simulink model "Test_N4"  (R2020b)
settings: Solver=ode3  StartTime=0.0  StopTime=inf  FixedStep=0.05  RelTol=1e-3
libraries: XBotBlockToolbox x3, Utilities x3

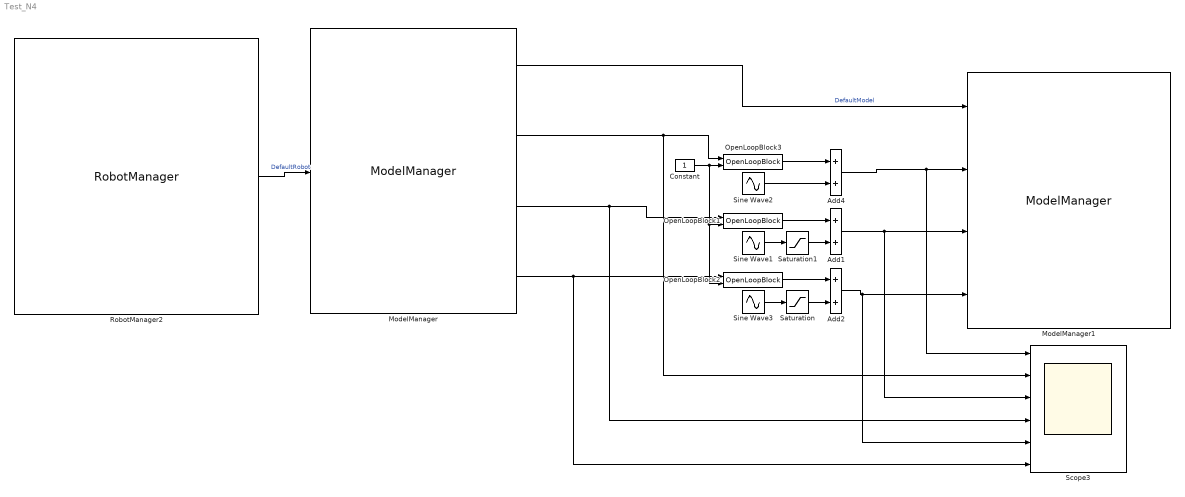
== system Test_N4 ==
  Add1 : Sum
  Add2 : Sum
  Add4 : Sum
  Constant : Constant
  ModelManager : XBotBlockToolbox/ModelManager  ModelName=DefaultModel  RobotName=DefaultRobot  UseExtModel=Off  SyncWithRobot=On  GetFloatingBaseList={}  SetFloatingBaseComponent=Off  GravityRequest=Off  ReadingsList={ 'qTemp', 'K', 'D' }  MechanicalLimitsList={}  MechanicalLimitsCheck=Off  MechanicalLimitsEnforce=Off  SensorList={}  ReferencesList={}  OldModelName=DefaultModel
  ModelManager1 : XBotBlockToolbox/ModelManager  ModelName=DefaultModel  RobotName=DefaultRobot  UseExtModel=On  SyncWithRobot=Off  GetFloatingBaseList={}  SetFloatingBaseComponent=Off  GravityRequest=Off  ReadingsList={}  MechanicalLimitsList={}  MechanicalLimitsCheck=Off  MechanicalLimitsEnforce=Off  SensorList={}  ReferencesList={ 'qTemp_ref', 'K_ref', 'D_ref' }  OldModelName=DefaultModel
  OpenLoopBlock1 : Utilities/OpenLoopBlock  SystemSampleTime=-1  VariantActivationTime=update diagram  Latency=0  AutoFrameSizeCalculation=off
  OpenLoopBlock2 : Utilities/OpenLoopBlock  SystemSampleTime=-1  VariantActivationTime=update diagram  Latency=0  AutoFrameSizeCalculation=off
  OpenLoopBlock3 : Utilities/OpenLoopBlock  SystemSampleTime=-1  VariantActivationTime=update diagram  Latency=0  AutoFrameSizeCalculation=off
  RobotManager2 : XBotBlockToolbox/RobotManager  RobotName=DefaultRobot  ModelName=DefaultModel  UseExtRobot=Off  SyncWithModel=Off  ReadingsList={}  MechanicalLimitsList={}  MechanicalLimitsCheck=Off  MechanicalLimitsEnforce=Off  SensorList={}  ReferencesList={}  OldRobotName=DefaultRobot
  Saturation : Saturate  UpperLimit=50  LowerLimit=0
  Saturation1 : Saturate  UpperLimit=1000  LowerLimit=0
  Scope3 : Scope  NumInputPorts=6
  Sine Wave1 : Sin  Amplitude=1000  SampleTime=0
  Sine Wave2 : Sin  Amplitude=50  SampleTime=0
  Sine Wave3 : Sin  Amplitude=50  SampleTime=0
  wires:
  OpenLoopBlock3/1 -> Add4/1
  Sine Wave2/1 -> Add4/2
  OpenLoopBlock1/1 -> Add1/1
  OpenLoopBlock2/1 -> Add2/1
  Add4/1 -> ModelManager1/2, Scope3/1
  Add1/1 -> ModelManager1/3, Scope3/3
  Add2/1 -> ModelManager1/4, Scope3/5
  Constant/1 -> OpenLoopBlock1/2, OpenLoopBlock2/2, OpenLoopBlock3/2
  ModelManager/2 -> Scope3/2, OpenLoopBlock3/1
  ModelManager/3 -> Scope3/4, OpenLoopBlock1/1
  ModelManager/4 -> Scope3/6, OpenLoopBlock2/1
  Saturation/1 -> Add2/2
  Sine Wave1/1 -> Saturation1/1
  Saturation1/1 -> Add1/2
  Sine Wave3/1 -> Saturation/1
  ModelManager/1 -> ModelManager1/1  "DefaultModel"
  RobotManager2/1 -> ModelManager/1  "DefaultRobot"
